simulink model "rigid_body_simulation"  (R2018b)
settings: Solver=ode5  StartTime=0.0  StopTime=10.0  FixedStep=0.02  MaxStep=0.02  RelTol=1e-3
InitFcn:
  | loadmatfile;
StopFcn:
  | rigid_body_plot;
libraries: shared6dof x1
settings Model: Creator=arthus  LastModifiedBy=arthus

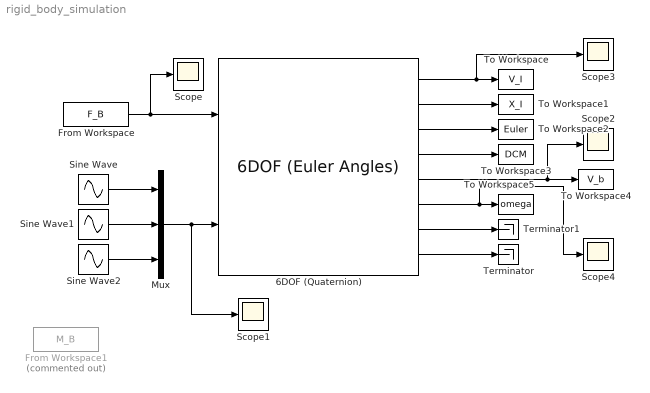
== system rigid_body_simulation ==
  6DOF (Quaternion) : shared6dof/6DOF (Euler Angles)  units=Metric (MKS)  mtype=Fixed  rep=Quaternion  xme_0=X_I  Vm_0=Vb_I  eul_0=Euler_I  pm_0=Omega_I  mass_0=1  mass_e=0.5  mass_f=2.0  inertia=diag([1 1 1])  inertia_e=eye(3)  inertia_f=2*eye(3)  k_quat=1.0  vre_flag=on  abi_flag=off  aMode=0  xme_statename=''  Vm_statename=''  eul_statename=''  quat_statename=''  pm_statename=''  mass_statename=''
      settings: SourceProductBaseCode=AE
  From Workspace : FromWorkspace  VariableName=F_B
  From Workspace1 : FromWorkspace  Commented=on  VariableName=M_B
  Mux : Mux  Inputs=3
  Scope{,1..4} (5 alike) : Scope
  Sine Wave : Sin  Frequency=pi  SampleTime=0
  Sine Wave1 : Sin  Frequency=pi  SampleTime=0
  Sine Wave2 : Sin  Frequency=pi  SampleTime=0
  Terminator : Terminator
  Terminator1 : Terminator
  To Workspace : ToWorkspace  VariableName=V_I  SampleTime=-1
  To Workspace1 : ToWorkspace  VariableName=X_I  SampleTime=-1
  To Workspace2 : ToWorkspace  VariableName=Euler  SampleTime=-1
  To Workspace3 : ToWorkspace  VariableName=DCM  SampleTime=-1
  To Workspace4 : ToWorkspace  VariableName=V_b  SampleTime=-1
  To Workspace5 : ToWorkspace  VariableName=omega  SampleTime=-1
  wires:
  From Workspace/1 -> Scope/1, 6DOF (Quaternion)/1
  6DOF (Quaternion)/1 -> Scope3/1, To Workspace/1
  6DOF (Quaternion)/2 -> To Workspace1/1
  6DOF (Quaternion)/3 -> To Workspace2/1
  6DOF (Quaternion)/4 -> To Workspace3/1
  6DOF (Quaternion)/5 -> Scope2/1, To Workspace4/1
  6DOF (Quaternion)/6 -> Scope4/1, To Workspace5/1
  6DOF (Quaternion)/7 -> Terminator1/1
  6DOF (Quaternion)/8 -> Terminator/1
  Mux/1 -> Scope1/1, 6DOF (Quaternion)/2
  Sine Wave/1 -> Mux/1
  Sine Wave1/1 -> Mux/2
  Sine Wave2/1 -> Mux/3
